simulink model "Dynamics_with_slip"  (R2020a)
settings: Solver=VariableStepAuto  StartTime=0.0  StopTime=10.0  RelTol=1e-3
values from neighbouring files (symbols this model uses):
  b = 0.05    [Dynamics_without_slip_test.m]    (also in Simulate_dynamics_with_slip.m)
  Iwy = 0.025    [Dynamics_without_slip_test.m]    (also in Simulate_dynamics_with_slip.m = 0.0025)
  Jeq = (I+2*Iwy*L^2/R^2)    (= 1.78127003695)    [Dynamics_without_slip_test.m]    (also in Simulate_dynamics_with_slip.m = 0.867793403695)
  K = 0.8    [Dynamics_without_slip_test.m]    (also in Simulate_dynamics_with_slip.m = 0.7)
  Ki = 12939e-3    (= 12.939)    [Simulate_dynamics_with_slip.m]
  Kv = Meq/0.8    (= 8.4671235358)    [Simulate_dynamics_with_slip.m]
  Kw = Jeq/0.8    (= 1.08474175462)    [Simulate_dynamics_with_slip.m]
  L = 0.164    [Dynamics_without_slip_test.m]    (also in Simulate_dynamics_with_slip.m)
  La = 0.088e-3    (= 8.8e-05)    [Simulate_dynamics_with_slip.m]
  mc = 2    [Dynamics_without_slip_test.m]    (also in Simulate_dynamics_with_slip.m)
  Meq = m+(2*Iwy/R^2)    (= 40.7369882864)    [Dynamics_without_slip_test.m]    (also in Simulate_dynamics_with_slip.m = 6.77369882864)
  mr = mc    (= 2)    [Dynamics_without_slip_test.m]    (also in Simulate_dynamics_with_slip.m)
  omega = v(:,2)    [Dynamics_without_slip_test.m]    (also in Simulate_dynamics_with_slip.m = 0; old_controller_modified.m = v(2))
  P1 = (Ic + 2*Iwy + L^2*mr + 4*b^2*mw + b^2*mr)    (= 0.845792)    [Dynamics_without_slip_test.m]    (also in Formulating_controller.m = (Ic + 2*Iwy + L^2*mr + 4*b^2*mw + b^2*mr); Simulate_dynamics_with_slip.m = 6.77369882864)
  P2 = (- mr*b^2 + mr*L^2 + Ic + 2*Iwy)    (= 0.830792)    [Dynamics_without_slip_test.m]    (also in Formulating_controller.m = -(- mr*b^2 + mr*L^2 + Ic + 2*Iwy); Simulate_dynamics_with_slip.m = 0.867793403695)
  r = 0.0364    [Simulate_dynamics_with_slip.m]
  Ra = 1.01    [Simulate_dynamics_with_slip.m]
  sat = 12    [Simulate_dynamics_with_slip.m]
  V = v(:,1)    [Dynamics_without_slip_test.m]    (also in Formulating_controller.m = 0.5*(ve^2+we^2); Simulate_dynamics_with_slip.m = 1; old_controller_modified.m = v(1))
libraries: simulink x3
settings Model: Creator=Omkar  LastModifiedBy=Omkar

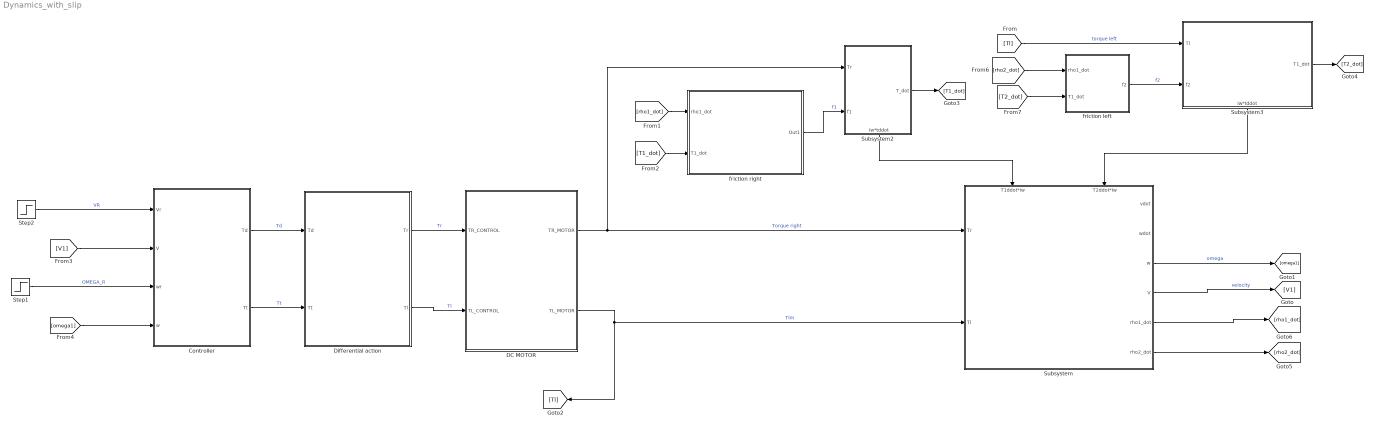
== system Dynamics_with_slip ==
  Controller : Subsystem
  DC MOTOR : Subsystem
      mask Display: image('D:\From open loop\Images\motor.jpg'); % Use "Edit Image" on toolstrip to change.
  Differential action : Subsystem
      mask Display: image('D:\From open loop\Images\diffg.jpg'); % Use "Edit Image" on toolstrip to change.
  Step1 : Step  After=omega  SampleTime=0
  Step2 : Step  After=V  SampleTime=0
  Subsystem : Subsystem
      settings: PortSchema="{\"entries\":[{\"content\":{\"sides\":[{\"content\":{\"connectorIds\":[\"In1\",\"In2\"]},\"type\":\"ConnectorPlacement.EquallySpacedRectSide\",\"uuid\":\"0f741662-0aa0-4f70-a7bc-4d81cf189765\"},{\"content\":{\"connectorIds\":[\"Out1\",\"Out2\",\"Out3\",\"Out4\",\"Out5\",\"Out6\"],\"side\":\"RIGHT\"},\"type\":\"ConnectorPlacement.EquallySpacedRectSide\",\"uuid\":\"61345bba-0f4e-4a45-813f-191783faa34f\"},{\"content\":{\"connectorIds\":[\"In3\",\"In4\"],\"side\":\"TOP\"},\"type\":\"ConnectorPlacement.EquallySpacedRectSide\",\"uuid\":\"0103c91a-592f-4929-b07b-fba43ce48b45\"}]},\"type\":\"ConnectorPlacement.EquallySpacedConnector\",\"uuid\":\"b6bd52cb-c94d-4866-979c-ba78b8ff4ad7\"}],\"packageUris\":[\"http://schema.mathworks.com/mf0/Connector/19700101\"],\"version\":\"1.0\"}"
  Subsystem2 : Subsystem
      settings: PortSchema="{\"entries\":[{\"content\":{\"sides\":[{\"content\":{\"connectorIds\":[]},\"type\":\"ConnectorPlacement.EquallySpacedRectSide\",\"uuid\":\"87b04e3d-c928-480c-a1a1-1313223c5e38\"},{\"content\":{\"connectorIds\":[\"Out1\"],\"side\":\"RIGHT\"},\"type\":\"ConnectorPlacement.EquallySpacedRectSide\",\"uuid\":\"24b15049-813d-4502-a6fe-723c7c9acef1\"},{\"content\":{\"connectorIds\":[\"In1\",\"In2\"],\"side\":\"TOP\"},\"type\":\"ConnectorPlacement.EquallySpacedRectSide\",\"uuid\":\"f1eb58bb-616f-4565-a8fb-035afd9aaf22\"},{\"content\":{\"connectorIds\":[\"Out2\"],\"side\":\"BOTTOM\"},\"type\":\"ConnectorPlacement.EquallySpacedRectSide\",\"uuid\":\"8c9ba54b-72de-4f17-9163-80eba6f391e2\"}]},\"type\":\"ConnectorPlacement.EquallySpacedConnector\",\"uuid\":\"ee8d76b6-d516-4cd3-af23-8bf5520b64c4\"}],\"packageUris\":[\"http://schema.mathworks.com/mf0/Connector/19700101\"],\"version\":\"1.0\"}"
  Subsystem3 : Subsystem
      settings: PortSchema="{\"entries\":[{\"content\":{\"sides\":[{\"content\":{\"connectorIds\":[]},\"type\":\"ConnectorPlacement.EquallySpacedRectSide\",\"uuid\":\"87b04e3d-c928-480c-a1a1-1313223c5e38\"},{\"content\":{\"connectorIds\":[\"Out1\"],\"side\":\"RIGHT\"},\"type\":\"ConnectorPlacement.EquallySpacedRectSide\",\"uuid\":\"24b15049-813d-4502-a6fe-723c7c9acef1\"},{\"content\":{\"connectorIds\":[\"In1\",\"In2\"],\"side\":\"TOP\"},\"type\":\"ConnectorPlacement.EquallySpacedRectSide\",\"uuid\":\"f1eb58bb-616f-4565-a8fb-035afd9aaf22\"},{\"content\":{\"connectorIds\":[\"Out2\"],\"side\":\"BOTTOM\"},\"type\":\"ConnectorPlacement.EquallySpacedRectSide\",\"uuid\":\"46d851b4-e0d9-4136-8fd7-44bf774a519f\"}]},\"type\":\"ConnectorPlacement.EquallySpacedConnector\",\"uuid\":\"ee8d76b6-d516-4cd3-af23-8bf5520b64c4\"}],\"packageUris\":[\"http://schema.mathworks.com/mf0/Connector/19700101\"],\"version\":\"1.0\"}"
  friction left : Subsystem
  friction right : Subsystem
  wires:
  Differential action/1(Tr) -> DC MOTOR/1(TR_CONTROL)  "Tr"
  DC MOTOR/2(TL_MOTOR) -> [Tl], Subsystem/2(Tl)  "Tlm"
  [omega1] -> Controller/4(w)
  Differential action/2(Tl) -> DC MOTOR/2(TL_CONTROL)  "Tl"
  Controller/1(Td) -> Differential action/1(Td)  "Td"
  Subsystem/4(V) -> [V1]  "velocity"
  Step2/1 -> Controller/1(Vr)  "VR"
  Step1/1 -> Controller/3(wr)  "OMEGA_R"
  Subsystem/3(w) -> [omega1]  "omega"
  Controller/2(Tt) -> Differential action/2(Tt)  "Tt"
  [V1] -> Controller/2(V)
  DC MOTOR/1(TR_MOTOR) -> Subsystem2/1(Tr), Subsystem/1(Tr)  "Torque right"
  Subsystem2/1(Iw*tddot) -> Subsystem/3(T1ddot*Iw)
  Subsystem3/1(Iw*tddot) -> Subsystem/4(T2ddot*Iw)
  [Tl] -> Subsystem3/1(Tl)  "torque left"
  Subsystem/6("rho2_dot ") -> [rho2_dot]
  Subsystem/5(rho1_dot) -> [rho1_dot]
  Subsystem3/2(T1_dot) -> [T2_dot]
  Subsystem2/2(T_dot) -> [T1_dot]
  [rho1_dot] -> friction right/1(rho1_dot)
  [T1_dot] -> friction right/2(T1_dot)
  friction right/1(Out1) -> Subsystem2/2(f1)  "f1"
  friction left/1(f2) -> Subsystem3/2(f2)  "f2"
  [rho2_dot] -> friction left/1(rho1_dot)
  [T2_dot] -> friction left/2(T1_dot)

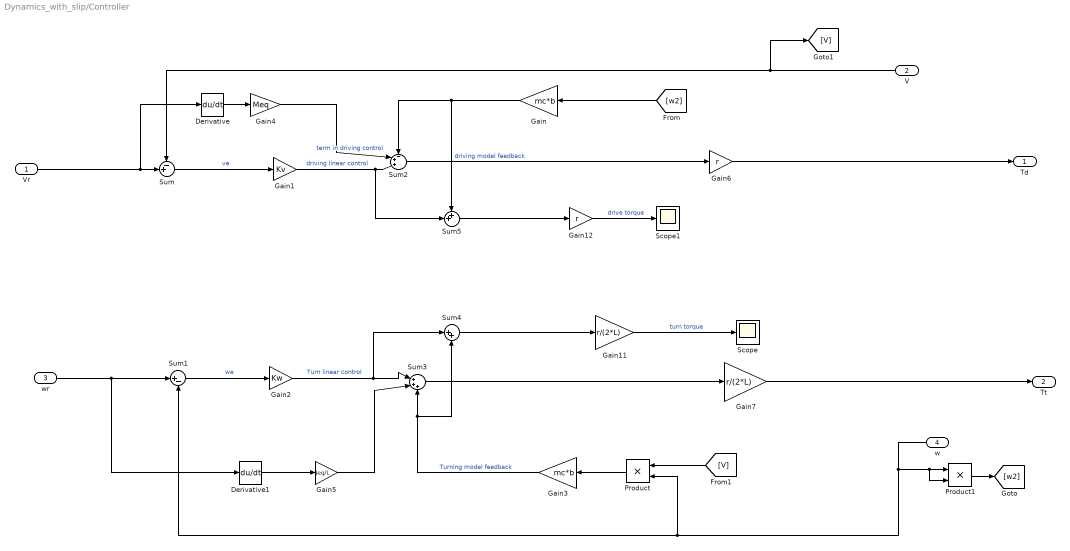
== system Dynamics_with_slip/Controller ==
  Vr : Inport
  V : Inport  Port=2
  wr : Inport  Port=3
  w : Inport  Port=4
  Derivative : Derivative
  Derivative1 : Derivative
  Gain : Gain  Gain=mc*b
  Gain1 : Gain  Gain=Kv
  Gain11 : Gain  Gain=r/(2*L)
  Gain12 : Gain  Gain=r
  Gain2 : Gain  Gain=Kw
  Gain3 : Gain  Gain=mc*b
  Gain4 : Gain  Gain=Meq
  Gain5 : Gain  Gain=Jeq/L
  Gain6 : Gain  Gain=r
  Gain7 : Gain  Gain=r/(2*L)
  Product : Product
  Product1 : Product
  Scope : Scope
  Scope1 : Scope
  Sum : Sum  Inputs=-+|
  Sum1 : Sum  Inputs=|+-
  Sum2 : Sum  Inputs=-++|
  Sum3 : Sum  Inputs=|+++
  Sum4 : Sum  Inputs=|++
  Sum5 : Sum  Inputs=++|
  Td : Outport
  Tt : Outport  Port=2
  wires:
  wr/1 -> Derivative1/1, Sum1/1
  Vr/1 -> Sum/2, Derivative/1
  V/1 -> Sum/1, [V]
  w/1 -> Product1/1, Product1/2, Product/2, Sum1/2
  [w2] -> Gain/1
  Gain/1 -> Sum5/1, Sum2/1  "driving model feedback"
  Gain1/1 -> Sum5/2, Sum2/3  "driving linear control"
  Sum/1 -> Gain1/1  "ve"
  Sum1/1 -> Gain2/1  "we"
  Gain2/1 -> Sum4/1, Sum3/1  "Turn linear control"
  [V] -> Product/1
  Product/1 -> Gain3/1
  Sum2/1 -> Gain6/1
  Product1/1 -> [w2]
  Sum3/1 -> Gain7/1
  Gain6/1 -> Td/1
  Derivative/1 -> Gain4/1
  Derivative1/1 -> Gain5/1
  Gain5/1 -> Sum3/2
  Gain7/1 -> Tt/1
  Gain3/1 -> Sum4/2, Sum3/3  "Turning model feedback"
  Sum4/1 -> Gain11/1
  Gain11/1 -> Scope/1  "turn torque"
  Sum5/1 -> Gain12/1
  Gain12/1 -> Scope1/1  "drive torque"
  Gain4/1 -> Sum2/2  "term in driving control"

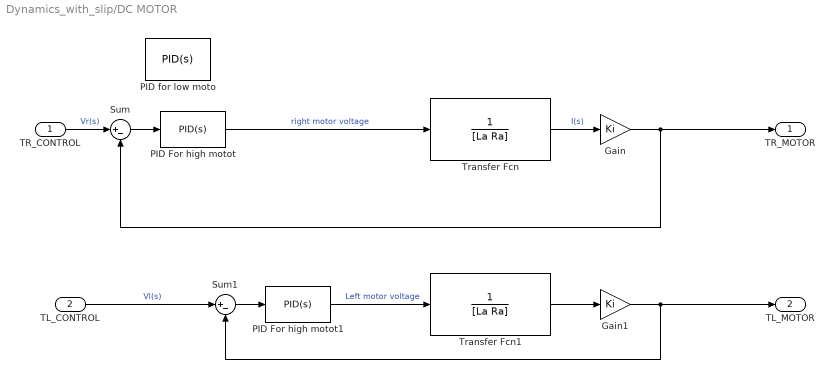
== system Dynamics_with_slip/DC MOTOR ==
  TR_CONTROL : Inport
  TL_CONTROL : Inport  Port=2
  Gain : Gain  Gain=Ki
  Gain1 : Gain  Gain=Ki
  PID For high motot : simulink/Continuous/PID Controller  Controller=PID  Form=Parallel  TimeDomain=Continuous-time  UseExternalTs=off  SampleTime=-1  IntegratorMethod=Forward Euler  FilterMethod=Forward Euler  ControllerParametersSource=internal  P=1.23021002052924  I=2  D=0.00945372952261552  UseFilter=on  N=100  TunerSelectOption=Transfer Function Based (PID Tuner App)  InitialConditionSource=internal  InitialConditionForIntegrator=0  InitialConditionForFilter=0  DifferentiatorICPrevScaledInput=0  ExternalReset=none  TrackingMode=off  Kt=1  LimitOutput=on  UpperSaturationLimit=12  LowerSaturationLimit=-12  LinearizeAsGain=off  AntiWindupMode=none  Kb=1  POutMin=[]  POutMax=[]  IOutMin=[]  IOutMax=[]  DOutMin=[]  DOutMax=[]  NOutMin=[]  NOutMax=[]  SumOutMin=[]  SumOutMax=[]  SaturationOutMin=[]  SaturationOutMax=[]  PParamMin=[]  PParamMax=[]  IParamMin=[]  IParamMax=[]  DParamMin=[]  DParamMax=[]  NParamMin=[]  NParamMax=[]  KbParamMin=[]  KbParamMax=[]  KtParamMin=[]  KtParamMax=[]  KbOutMin=[]  KbOutMax=[]  KtOutMin=[]  KtOutMax=[]  IntegratorOutMin=[]  IntegratorOutMax=[]  FilterOutMin=[]  FilterOutMax=[]  SumI1OutMin=[]  SumI1OutMax=[]  SumI2OutMin=[]  SumI2OutMax=[]  SumI3OutMin=[]  SumI3OutMax=[]  SumI4OutMin=[]  SumI4OutMax=[]  SumDOutMin=[]  SumDOutMax=[]  DifferentiatorOutMin=[]  DifferentiatorOutMax=[]  FilterDiffOutCoefMin=[]  FilterDiffOutCoefMax=[]  ReciprocalOutMin=[]  ReciprocalOutMax=[]  SumDenOutMin=[]  SumDenOutMax=[]  SumNumOutMin=[]  SumNumOutMax=[]  DivideOutMin=[]  DivideOutMax=[]  UdiffTsProdOutMin=[]  UdiffTsProdOutMax=[]  NTsProdOutMin=[]  NTsProdOutMax=[]  UintegralTsProdOutMin=[]  UintegralTsProdOutMax=[]  UngainTsProdOutMin=[]  UngainTsProdOutMax=[]  IntegratorContinuousStateAttributes=''  IntegratorStateMustResolveToSignalObject=off  IntegratorRTWStateStorageClass=Auto  FilterContinuousStateAttributes=''  FilterStateMustResolveToSignalObject=off  FilterRTWStateStorageClass=Auto  ParallelPVariant=InternalParameters  IdealPVariant=Disabled  IVariant=InternalParameters  DVariant=InternalParameters  IntegratorVariant=Continuous  SatVariant=Enabled  AWVariant=Passthrough  PCopyVariant=Disabled  TRVariant=Disabled  FdbkBlocksVariant=Forward  IdealPFdbkVariant=Disabled  SatFdbkVariant=Disabled  DerivativeFilterVariant=ContFilter  NVariant=InternalParameters  NCopyVariant=Disabled  FilterICVariant=InternalICsFilter  IntegratorICVariant=InternalICs  ExternalResetVariant=Disabled  TRSumVariant=Passthrough  SumFdbkVariant=Disabled  SumVariant=Sum_PID  TsampFilterVariant=InternalTs  TsampNgainVariant=Passthrough  TsampIntegralVariant=Passthrough
  PID For high motot1 : simulink/Continuous/PID Controller  Controller=PID  Form=Parallel  TimeDomain=Continuous-time  UseExternalTs=off  SampleTime=-1  IntegratorMethod=Forward Euler  FilterMethod=Forward Euler  ControllerParametersSource=internal  P=1.23021002052924  I=2  D=0.00945372952261552  UseFilter=on  N=100  TunerSelectOption=Transfer Function Based (PID Tuner App)  InitialConditionSource=internal  InitialConditionForIntegrator=0  InitialConditionForFilter=0  DifferentiatorICPrevScaledInput=0  ExternalReset=none  TrackingMode=off  Kt=1  LimitOutput=on  UpperSaturationLimit=12  LowerSaturationLimit=-12  LinearizeAsGain=off  AntiWindupMode=none  Kb=1  POutMin=[]  POutMax=[]  IOutMin=[]  IOutMax=[]  DOutMin=[]  DOutMax=[]  NOutMin=[]  NOutMax=[]  SumOutMin=[]  SumOutMax=[]  SaturationOutMin=[]  SaturationOutMax=[]  PParamMin=[]  PParamMax=[]  IParamMin=[]  IParamMax=[]  DParamMin=[]  DParamMax=[]  NParamMin=[]  NParamMax=[]  KbParamMin=[]  KbParamMax=[]  KtParamMin=[]  KtParamMax=[]  KbOutMin=[]  KbOutMax=[]  KtOutMin=[]  KtOutMax=[]  IntegratorOutMin=[]  IntegratorOutMax=[]  FilterOutMin=[]  FilterOutMax=[]  SumI1OutMin=[]  SumI1OutMax=[]  SumI2OutMin=[]  SumI2OutMax=[]  SumI3OutMin=[]  SumI3OutMax=[]  SumI4OutMin=[]  SumI4OutMax=[]  SumDOutMin=[]  SumDOutMax=[]  DifferentiatorOutMin=[]  DifferentiatorOutMax=[]  FilterDiffOutCoefMin=[]  FilterDiffOutCoefMax=[]  ReciprocalOutMin=[]  ReciprocalOutMax=[]  SumDenOutMin=[]  SumDenOutMax=[]  SumNumOutMin=[]  SumNumOutMax=[]  DivideOutMin=[]  DivideOutMax=[]  UdiffTsProdOutMin=[]  UdiffTsProdOutMax=[]  NTsProdOutMin=[]  NTsProdOutMax=[]  UintegralTsProdOutMin=[]  UintegralTsProdOutMax=[]  UngainTsProdOutMin=[]  UngainTsProdOutMax=[]  IntegratorContinuousStateAttributes=''  IntegratorStateMustResolveToSignalObject=off  IntegratorRTWStateStorageClass=Auto  FilterContinuousStateAttributes=''  FilterStateMustResolveToSignalObject=off  FilterRTWStateStorageClass=Auto  ParallelPVariant=InternalParameters  IdealPVariant=Disabled  IVariant=InternalParameters  DVariant=InternalParameters  IntegratorVariant=Continuous  SatVariant=Enabled  AWVariant=Passthrough  PCopyVariant=Disabled  TRVariant=Disabled  FdbkBlocksVariant=Forward  IdealPFdbkVariant=Disabled  SatFdbkVariant=Disabled  DerivativeFilterVariant=ContFilter  NVariant=InternalParameters  NCopyVariant=Disabled  FilterICVariant=InternalICsFilter  IntegratorICVariant=InternalICs  ExternalResetVariant=Disabled  TRSumVariant=Passthrough  SumFdbkVariant=Disabled  SumVariant=Sum_PID  TsampFilterVariant=InternalTs  TsampNgainVariant=Passthrough  TsampIntegralVariant=Passthrough
  PID for low moto : simulink/Continuous/PID Controller  Controller=PID  Form=Parallel  TimeDomain=Continuous-time  UseExternalTs=off  SampleTime=-1  IntegratorMethod=Forward Euler  FilterMethod=Forward Euler  ControllerParametersSource=internal  P=274.861697101044  I=555.220628144108  D=0  UseFilter=on  N=100  TunerSelectOption=Transfer Function Based (PID Tuner App)  InitialConditionSource=internal  InitialConditionForIntegrator=0  InitialConditionForFilter=0  DifferentiatorICPrevScaledInput=0  ExternalReset=none  TrackingMode=off  Kt=1  LimitOutput=on  UpperSaturationLimit=sat  LowerSaturationLimit=-sat  LinearizeAsGain=off  AntiWindupMode=back-calculation  Kb=1  POutMin=[]  POutMax=[]  IOutMin=[]  IOutMax=[]  DOutMin=[]  DOutMax=[]  NOutMin=[]  NOutMax=[]  SumOutMin=[]  SumOutMax=[]  SaturationOutMin=[]  SaturationOutMax=[]  PParamMin=[]  PParamMax=[]  IParamMin=[]  IParamMax=[]  DParamMin=[]  DParamMax=[]  NParamMin=[]  NParamMax=[]  KbParamMin=[]  KbParamMax=[]  KtParamMin=[]  KtParamMax=[]  KbOutMin=[]  KbOutMax=[]  KtOutMin=[]  KtOutMax=[]  IntegratorOutMin=[]  IntegratorOutMax=[]  FilterOutMin=[]  FilterOutMax=[]  SumI1OutMin=[]  SumI1OutMax=[]  SumI2OutMin=[]  SumI2OutMax=[]  SumI3OutMin=[]  SumI3OutMax=[]  SumI4OutMin=[]  SumI4OutMax=[]  SumDOutMin=[]  SumDOutMax=[]  DifferentiatorOutMin=[]  DifferentiatorOutMax=[]  FilterDiffOutCoefMin=[]  FilterDiffOutCoefMax=[]  ReciprocalOutMin=[]  ReciprocalOutMax=[]  SumDenOutMin=[]  SumDenOutMax=[]  SumNumOutMin=[]  SumNumOutMax=[]  DivideOutMin=[]  DivideOutMax=[]  UdiffTsProdOutMin=[]  UdiffTsProdOutMax=[]  NTsProdOutMin=[]  NTsProdOutMax=[]  UintegralTsProdOutMin=[]  UintegralTsProdOutMax=[]  UngainTsProdOutMin=[]  UngainTsProdOutMax=[]  IntegratorContinuousStateAttributes=''  IntegratorStateMustResolveToSignalObject=off  IntegratorRTWStateStorageClass=Auto  FilterContinuousStateAttributes=''  FilterStateMustResolveToSignalObject=off  FilterRTWStateStorageClass=Auto  ParallelPVariant=InternalParameters  IdealPVariant=Disabled  IVariant=InternalParameters  DVariant=InternalParameters  IntegratorVariant=Continuous  SatVariant=Enabled  AWVariant=BackCalculation  PCopyVariant=Disabled  TRVariant=Disabled  FdbkBlocksVariant=Forward  IdealPFdbkVariant=Disabled  SatFdbkVariant=Disabled  DerivativeFilterVariant=ContFilter  NVariant=InternalParameters  NCopyVariant=Disabled  FilterICVariant=InternalICsFilter  IntegratorICVariant=InternalICs  ExternalResetVariant=Disabled  TRSumVariant=Passthrough  SumFdbkVariant=Disabled  SumVariant=Sum_PID  TsampFilterVariant=InternalTs  TsampNgainVariant=Passthrough  TsampIntegralVariant=Passthrough
  Sum : Sum  Inputs=|+-
  Sum1 : Sum  Inputs=|+-
  Transfer Fcn : TransferFcn  Denominator=[La Ra]
  Transfer Fcn1 : TransferFcn  Denominator=[La Ra]
  TR_MOTOR : Outport
  TL_MOTOR : Outport  Port=2
  wires:
  Gain/1 -> TR_MOTOR/1, Sum/2
  Transfer Fcn/1 -> Gain/1  "I(s)"
  TR_CONTROL/1 -> Sum/1  "Vr(s)"
  Sum/1 -> PID For high motot/1
  TL_CONTROL/1 -> Sum1/1  "Vl(s)"
  Sum1/1 -> PID For high motot1/1
  Transfer Fcn1/1 -> Gain1/1
  Gain1/1 -> TL_MOTOR/1, Sum1/2
  PID For high motot/1 -> Transfer Fcn/1  "right motor voltage"
  PID For high motot1/1 -> Transfer Fcn1/1  "Left motor voltage"

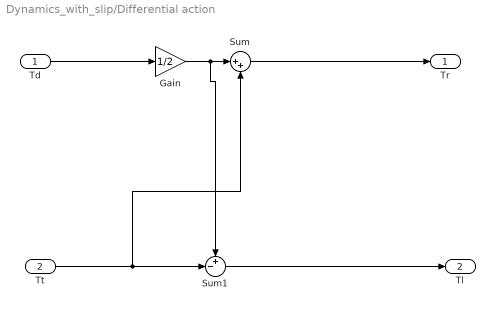
== system Dynamics_with_slip/Differential action ==
  Td : Inport
  Tt : Inport  Port=2
  Gain : Gain  Gain=1/2
  Sum : Sum  Inputs=|++
  Sum1 : Sum  Inputs=+-|
  Tr : Outport
  Tl : Outport  Port=2
  wires:
  Tt/1 -> Sum1/2, Sum/2
  Td/1 -> Gain/1
  Sum/1 -> Tr/1
  Sum1/1 -> Tl/1
  Gain/1 -> Sum1/1, Sum/1

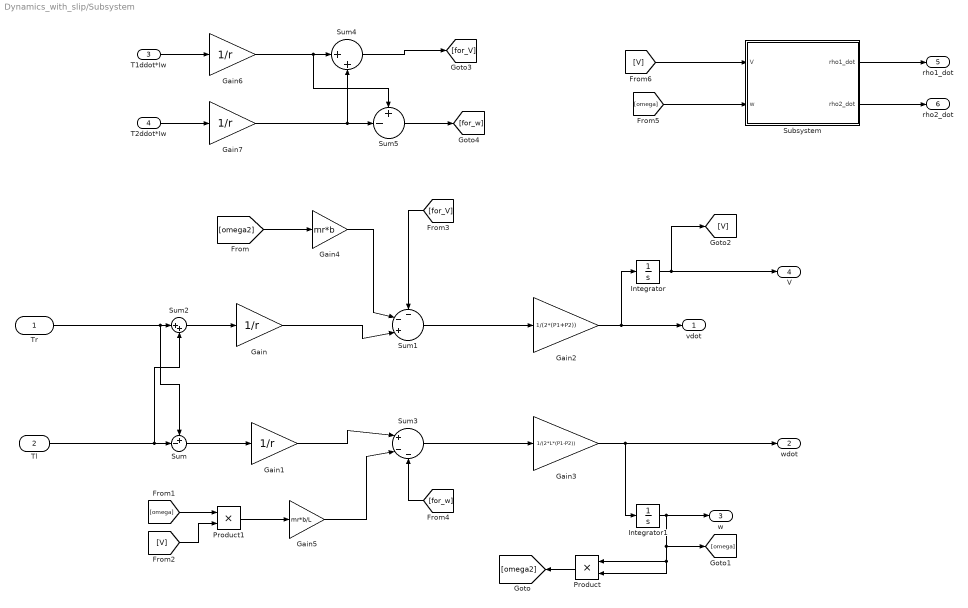
== system Dynamics_with_slip/Subsystem ==
  Tr : Inport
  Tl : Inport  Port=2
  T1ddot*Iw : Inport  Port=3
  T2ddot*Iw : Inport  Port=4
  Gain{,1,6..7} (4 alike) : Gain  Gain=1/r
  Gain2 : Gain  Gain=1/(2*(P1+P2))
  Gain3 : Gain  Gain=1/(2*L*(P1-P2))
  Gain4 : Gain  Gain=mr*b
  Gain5 : Gain  Gain=mr*b/L
  Integrator : Integrator
  Integrator1 : Integrator
  Product : Product
  Product1 : Product
  Subsystem : Subsystem
  Sum : Sum  Inputs=+-|
  Sum1 : Sum  Inputs=--+|
  Sum2 : Sum  Inputs=|++
  Sum3 : Sum  Inputs=|+--
  Sum4 : Sum  Inputs=|++
  Sum5 : Sum  Inputs=+-|
  vdot : Outport
  wdot : Outport  Port=2
  w : Outport  Port=3
  V : Outport  Port=4
  rho1_dot : Outport  Port=5
  "rho2_dot " : Outport  Port=6
  wires:
  Tr/1 -> Sum/1, Sum2/1
  Tl/1 -> Sum/2, Sum2/2
  Sum2/1 -> Gain/1
  Sum/1 -> Gain1/1
  Gain3/1 -> Integrator1/1, wdot/1
  Gain2/1 -> Integrator/1, vdot/1
  Integrator/1 -> [V], V/1
  Integrator1/1 -> [omega], Product/1, Product/2, w/1
  Product/1 -> [omega2]
  [omega2] -> Gain4/1
  Gain/1 -> Sum1/3
  Gain4/1 -> Sum1/2
  Gain1/1 -> Sum3/1
  Gain5/1 -> Sum3/2
  Product1/1 -> Gain5/1
  [omega] -> Product1/1
  [V] -> Product1/2
  T1ddot*Iw/1 -> Gain6/1
  T2ddot*Iw/1 -> Gain7/1
  Gain6/1 -> Sum5/1, Sum4/1
  Gain7/1 -> Sum5/2, Sum4/2
  Sum4/1 -> [for_V]
  Sum5/1 -> [for_w]
  [for_V] -> Sum1/1
  Sum1/1 -> Gain2/1
  [for_w] -> Sum3/3
  Sum3/1 -> Gain3/1
  [V] -> Subsystem/1(V)
  [omega] -> Subsystem/2(w)
  Subsystem/1(rho1_dot) -> rho1_dot/1
  Subsystem/2("rho2_dot ") -> "rho2_dot "/1

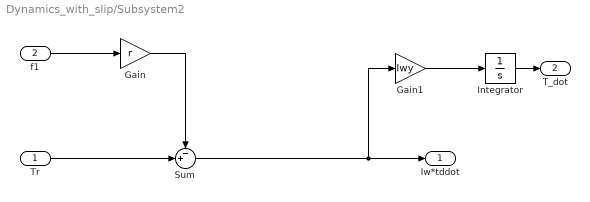
== system Dynamics_with_slip/Subsystem2 ==
  Tr : Inport
  f1 : Inport  Port=2
  Gain : Gain  Gain=r
  Gain1 : Gain  Gain=Iwy
  Integrator : Integrator
  Sum : Sum  Inputs=-+|
  Iw*tddot : Outport
  T_dot : Outport  Port=2
  wires:
  Tr/1 -> Sum/2
  Gain/1 -> Sum/1
  f1/1 -> Gain/1
  Integrator/1 -> T_dot/1
  Sum/1 -> Gain1/1, Iw*tddot/1
  Gain1/1 -> Integrator/1

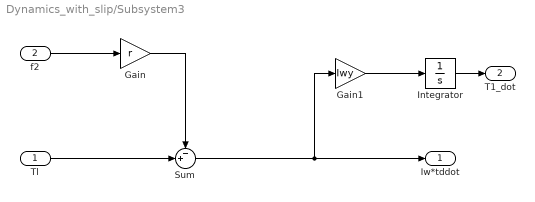
== system Dynamics_with_slip/Subsystem3 ==
  Tl : Inport
  f2 : Inport  Port=2
  Gain : Gain  Gain=r
  Gain1 : Gain  Gain=Iwy
  Integrator : Integrator
  Sum : Sum  Inputs=-+|
  Iw*tddot : Outport
  T1_dot : Outport  Port=2
  wires:
  Tl/1 -> Sum/2
  Gain/1 -> Sum/1
  f2/1 -> Gain/1
  Sum/1 -> Gain1/1, Iw*tddot/1
  Integrator/1 -> T1_dot/1
  Gain1/1 -> Integrator/1

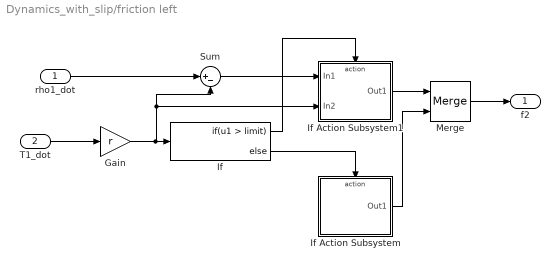
== system Dynamics_with_slip/friction left ==
  rho1_dot : Inport
  T1_dot : Inport  Port=2
  Gain : Gain  Gain=r
  If : If  IfExpression=u1 > limit
  If Action Subsystem : Subsystem  TreatAsAtomicUnit=on
  If Action Subsystem1 : Subsystem  TreatAsAtomicUnit=on
  Merge : Merge
  Sum : Sum  Inputs=|+-
  f2 : Outport
  wires:
  Merge/1 -> f2/1
  T1_dot/1 -> Gain/1
  If Action Subsystem/1(Out1) -> Merge/2
  If Action Subsystem1/1(Out1) -> Merge/1
  rho1_dot/1 -> Sum/1
  Sum/1 -> If Action Subsystem1/1(In1)
  If/1 -> If Action Subsystem1/Action
  If/2 -> If Action Subsystem/Action
  Gain/1 -> Sum/2, If Action Subsystem1/2(In2), If/1

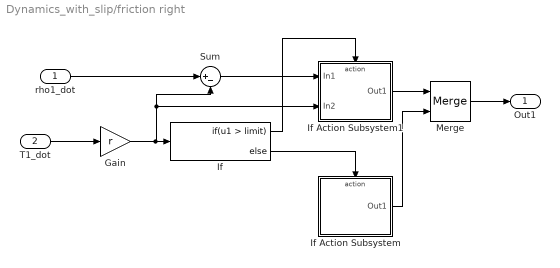
== system Dynamics_with_slip/friction right ==
  rho1_dot : Inport
  T1_dot : Inport  Port=2
  Gain : Gain  Gain=r
  If : If  IfExpression=u1 > limit
  If Action Subsystem : Subsystem  TreatAsAtomicUnit=on
  If Action Subsystem1 : Subsystem  TreatAsAtomicUnit=on
  Merge : Merge
  Sum : Sum  Inputs=|+-
  Out1 : Outport
  wires:
  Merge/1 -> Out1/1
  T1_dot/1 -> Gain/1
  If Action Subsystem/1(Out1) -> Merge/2
  If Action Subsystem1/1(Out1) -> Merge/1
  rho1_dot/1 -> Sum/1
  Sum/1 -> If Action Subsystem1/1(In1)
  If/1 -> If Action Subsystem1/Action
  If/2 -> If Action Subsystem/Action
  Gain/1 -> Sum/2, If Action Subsystem1/2(In2), If/1

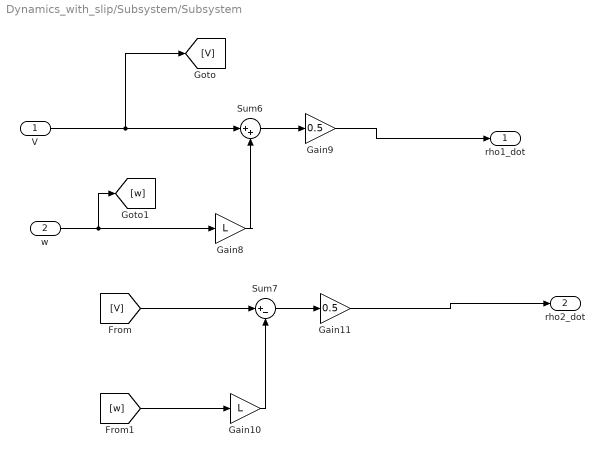
== system Dynamics_with_slip/Subsystem/Subsystem ==
  V : Inport
  w : Inport  Port=2
  Gain10 : Gain  Gain=L
  Gain11 : Gain  Gain=0.5
  Gain8 : Gain  Gain=L
  Gain9 : Gain  Gain=0.5
  Sum6 : Sum  Inputs=|++
  Sum7 : Sum  Inputs=|+-
  rho1_dot : Outport
  "rho2_dot " : Outport  Port=2
  wires:
  Gain11/1 -> "rho2_dot "/1
  Gain9/1 -> rho1_dot/1
  V/1 -> [V], Sum6/1
  Gain8/1 -> Sum6/2
  Sum6/1 -> Gain9/1
  Sum7/1 -> Gain11/1
  Gain10/1 -> Sum7/2
  [w] -> Gain10/1
  w/1 -> [w], Gain8/1
  [V] -> Sum7/1

== system Dynamics_with_slip/friction left/If Action Subsystem ==
  Action Port : ActionPort  ActionPortLabel=else
  Zero : Constant  Value=0  OutDataTypeStr=Inherit: Inherit via back propagation
  Out1 : Outport
  wires:
  Zero/1 -> Out1/1

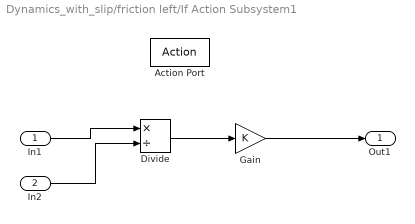
== system Dynamics_with_slip/friction left/If Action Subsystem1 ==
  In1 : Inport
  In2 : Inport  Port=2
  Action Port : ActionPort  ActionPortLabel=if(u1 > limit)
  Divide : Product  Inputs=*/  RndMeth=Zero  SaturateOnIntegerOverflow=on
  Gain : Gain  Gain=K
  Out1 : Outport
  wires:
  In1/1 -> Divide/1
  In2/1 -> Divide/2
  Divide/1 -> Gain/1
  Gain/1 -> Out1/1

== system Dynamics_with_slip/friction right/If Action Subsystem ==
  Action Port : ActionPort  ActionPortLabel=else
  Zero : Constant  Value=0  OutDataTypeStr=Inherit: Inherit via back propagation
  Out1 : Outport
  wires:
  Zero/1 -> Out1/1

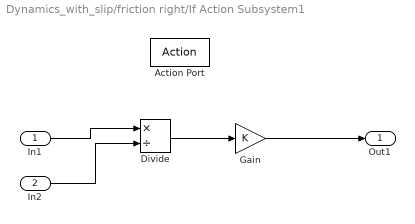
== system Dynamics_with_slip/friction right/If Action Subsystem1 ==
  In1 : Inport
  In2 : Inport  Port=2
  Action Port : ActionPort  ActionPortLabel=if(u1 > limit)
  Divide : Product  Inputs=*/  RndMeth=Zero  SaturateOnIntegerOverflow=on
  Gain : Gain  Gain=K
  Out1 : Outport
  wires:
  In1/1 -> Divide/1
  In2/1 -> Divide/2
  Divide/1 -> Gain/1
  Gain/1 -> Out1/1
